simulink library "hbtc"  (Simulink 8.1)
settings: Solver=ode1  StartTime=0.0  StopTime=Inf  FixedStep=0.001  RelTol=1e-3
PostLoadFcn:
  | , if any(exist('dsrtsu_mdlpostloadfcn', 'file') == [2, 3, 6]), try dsrtsu_mdlpostloadfcn('Execute', bdroot); catch fprintf('Error in PostLoadFcn (dsrtsu_mdlpostloadfcn) for model "%s":\n %s\n', bdroot, lasterr); end, end,
settings Model: DSRTSU_INTERNAL_RTI_VER=450  DSRTSU_INTERNAL_RTI_TYPE=rti1401  Creator=tescamilla  LastModifiedBy=tescamilla

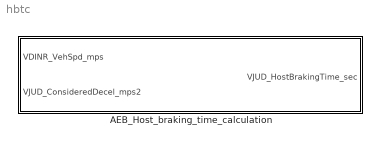
== system hbtc ==
  AEB_Host_braking_time_calculation : Subsystem

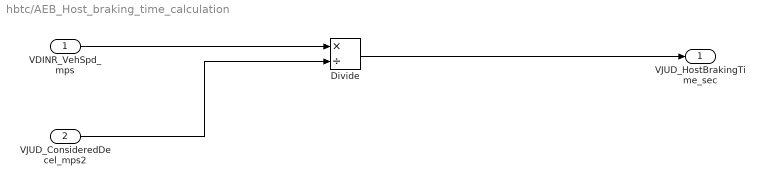
== system hbtc/AEB_Host_braking_time_calculation ==
  VDINR_VehSpd_mps : Inport
  VJUD_ConsideredDecel_mps2 : Inport  Port=2
  Divide : Product  Inputs=*/
  VJUD_HostBrakingTime_sec : Outport
  wires:
  Divide/1 -> VJUD_HostBrakingTime_sec/1
  VDINR_VehSpd_mps/1 -> Divide/1
  VJUD_ConsideredDecel_mps2/1 -> Divide/2
